simulink model "second"  (R2022b)
settings: Solver=VariableStepAuto  StartTime=0.0  StopTime=10.0  RelTol=1e-3
libraries: spsIGBTDiodeLib x5, simulink x4, spsSeriesRLCBranchLib x4, spsCurrentMeasurementLib x2, spsGroundLib x2, spsVoltageMeasurementLib x2, spsACVoltageSourceLib x1, spsDiodeLib x1, spsPVArrayLib x1, spspowerguiLib x1
settings Model: Creator=Xheng  LastModifiedBy=Xheng

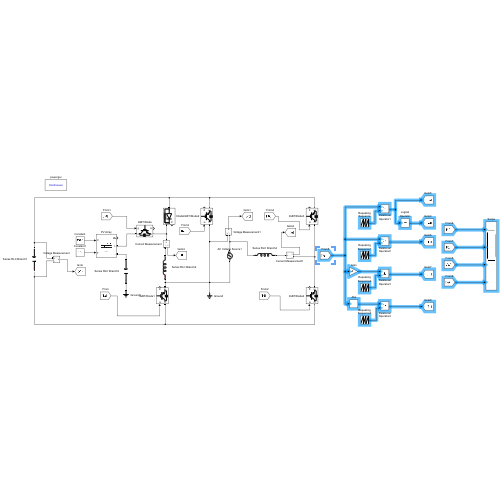
[thumbnail: Simulink's stored preview of the top-level diagram]
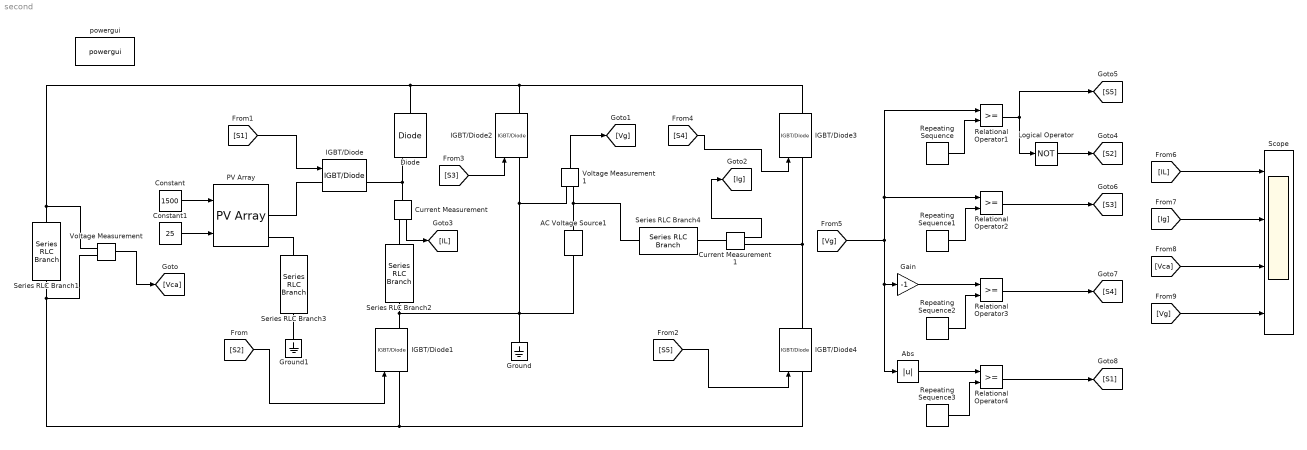
== system second ==
  AC Voltage Source1 : spsACVoltageSourceLib/AC Voltage Source  Amplitude=100  Phase=0  Frequency=60  SampleTime=0  Measurements=None  BusType=swing  Pref=10e3  Qref=0  Qmin=-inf  Qmax=+inf
  Abs : Abs  SaturateOnIntegerOverflow=off
  Constant : Constant  Value=1500
  Constant1 : Constant  Value=25
  Current Measurement : spsCurrentMeasurementLib/Current Measurement  PhasorSimulation=off  OutputType=Complex  PSBequivalent=0
  Current Measurement1 : spsCurrentMeasurementLib/Current Measurement  PhasorSimulation=off  OutputType=Complex  PSBequivalent=0
  Diode : spsDiodeLib/Diode  Ron=0.001  Lon=0  Vf=0.8  IC=0  UseSnubber=0  Rs=500  Cs=250e-9  Measurements=on
  Gain : Gain  Gain=-1
  Ground : spsGroundLib/Ground  LConnTagsString=a
  Ground1 : spsGroundLib/Ground  LConnTagsString=a
  IGBT/Diode{,1..4} (5 alike) : spsIGBTDiodeLib/IGBT//Diode  Ron=1e-3  Rs=1e5  Cs=inf  Measurements=on
  Logical Operator : Logic  Operator=NOT  AllPortsSameDT=off  OutDataTypeStr=boolean
  PV Array : spsPVArrayLib/PV Array  Npar=40  Nser=10  PlotType=array @ 1000 W/m2 & specified temperatures  S_vec="[ 1000  500  100 ]"  Temp_C_vec="[ 45 25  ]"  ModuleName=User-defined  PlotWhenSelected=off  Pm=213.15  Ncell=60  Voc=36.3  Isc=7.84  Vm=29  Im=7.35  beta_Voc_pc=-0.36099  alpha_Isc_pc=0.102  beta_Voc=-0.13104  alpha_Isc=0.0079968  IL=7.8654  I0=2.9273e-10  nI=0.98119  Rsh=313.0553  Rs=0.39381  RobustModel=off  RobustCellTemperature=313.3991  BAL=on  Tc=1e-6  Tfilter=5e-5
  Relational Operator{1..4} (4 alike) : RelationalOperator  OutDataTypeStr=boolean  RndMeth=Simplest  InputSameDT=off
  Repeating Sequence{,1..3} (4 alike) : simulink/Sources/Repeating Sequence  rep_seq_t=[0 2]  rep_seq_y=[0 2]
  Scope : Scope  NumInputPorts=4
  Series RLC Branch1 : spsSeriesRLCBranchLib/Series RLC Branch  LConnTagsString=__new0  RConnTagsString=__new0  BranchType=C  Resistance=1  Inductance=1e-3  SetiL0=off  InitialCurrent=0  Capacitance=50e-6  Setx0=off  InitialVoltage=0  Measurements=None
  Series RLC Branch2 : spsSeriesRLCBranchLib/Series RLC Branch  LConnTagsString=__new0  RConnTagsString=__new0  BranchType=L  Resistance=1  Inductance=115e-6  SetiL0=off  InitialCurrent=0  Capacitance=1e-6  Setx0=off  InitialVoltage=0  Measurements=None
  Series RLC Branch3 : spsSeriesRLCBranchLib/Series RLC Branch  LConnTagsString=__new0  RConnTagsString=__new0  BranchType=C  Resistance=1  Inductance=1e-3  SetiL0=off  InitialCurrent=0  Capacitance=50e-6  Setx0=off  InitialVoltage=0  Measurements=None
  Series RLC Branch4 : spsSeriesRLCBranchLib/Series RLC Branch  LConnTagsString=__new0  RConnTagsString=__new0  BranchType=L  Resistance=1  Inductance=115e-6  SetiL0=off  InitialCurrent=0  Capacitance=1e-6  Setx0=off  InitialVoltage=0  Measurements=None
  Voltage Measurement : spsVoltageMeasurementLib/Voltage Measurement  PhasorSimulation=off  OutputType=Complex  PSBequivalent=0
  Voltage Measurement1 : spsVoltageMeasurementLib/Voltage Measurement  PhasorSimulation=off  OutputType=Complex  PSBequivalent=0
  powergui : spspowerguiLib/powergui  Priority=1  SimulationMode=Continuous  SampleTime=50e-6  frequency=60  Iterations=50  frequencyindice=60  Pbase=100e6  ErrMax=1e-4  UnitsV=kV  UnitsW=MW  buscounter=0  FunctionMessages=off  echomessages=off  EnableUseOfTLC=off  CurrentSourceSwitches=off  DisableSnubberDevices=off  DisableRonSwitches=off  DisableVfSwitches=off  DisplayEquations=off  AutomaticDiscreteSolvers=off  SolverType=Tustin/Backward Euler (TBE)  Interpol=off  ExternalGateDelay=off  methode=off  Ts=100  x0status=blocks  SPID=on  SwTol=0  HookPort=off  NonlinearTolerance=1e-4  nMaxIteration=100  ContinueOnMaxIteration=off  RestoreLinks=warning  ResistiveCurrentMeasurement=off  Frange=[0:2:500]  Ylog=off  Xlog=on  ShowGrid=off  save=off  variable=ZData  structure=0  ZoomFFT=off  StartTime=0.0  cycles=1  DisplayStyle=1  fundamental=60  FreqAxis=off  MaxFrequency=1000  frequencyindicesteady=1  RmsSteady=1  display=off
  wires:
  Constant1/1 -> PV Array/2
  Constant/1 -> PV Array/1
  Voltage Measurement/1 -> [Vca]
  Voltage Measurement1/1 -> [Vg]
  Current Measurement1/1 -> [Ig]
  Current Measurement/1 -> [IL]
  [S1] -> IGBT/Diode/1
  [S2] -> IGBT/Diode1/1
  [S5] -> IGBT/Diode4/1
  [S3] -> IGBT/Diode2/1
  [S4] -> IGBT/Diode3/1
  Logical Operator/1 -> [S2]
  Relational Operator1/1 -> Logical Operator/1, [S5]
  [Vg] -> Abs/1, Gain/1, Relational Operator1/1, Relational Operator2/1
  Repeating Sequence/1 -> Relational Operator1/2
  Repeating Sequence1/1 -> Relational Operator2/2
  Relational Operator2/1 -> [S3]
  Repeating Sequence2/1 -> Relational Operator3/2
  Relational Operator3/1 -> [S4]
  Repeating Sequence3/1 -> Relational Operator4/2
  Relational Operator4/1 -> [S1]
  Gain/1 -> Relational Operator3/1
  Abs/1 -> Relational Operator4/1
  [IL] -> Scope/1
  [Ig] -> Scope/2
  [Vca] -> Scope/3
  [Vg] -> Scope/4
  connections:
  PV Array/RConn1 -- IGBT/Diode/LConn1
  IGBT/Diode/RConn1 -- Diode/RConn1 -- Current Measurement/LConn1
  Diode/LConn1 -- IGBT/Diode3/RConn1 -- IGBT/Diode2/RConn1 -- Voltage Measurement/LConn1 -- Series RLC Branch1/RConn1
  Voltage Measurement/LConn2 -- IGBT/Diode1/LConn1 -- IGBT/Diode4/LConn1 -- Series RLC Branch1/LConn1
  Current Measurement/RConn1 -- Series RLC Branch2/RConn1
  Series RLC Branch2/LConn1 -- Voltage Measurement1/LConn1 -- IGBT/Diode2/LConn1 -- Ground/LConn1 -- AC Voltage Source1/LConn1 -- IGBT/Diode1/RConn1
  PV Array/RConn2 -- Series RLC Branch3/RConn1
  Current Measurement1/LConn1 -- Series RLC Branch4/RConn1
  Current Measurement1/RConn1 -- IGBT/Diode3/LConn1 -- IGBT/Diode4/RConn1
  AC Voltage Source1/RConn1 -- Series RLC Branch4/LConn1 -- Voltage Measurement1/LConn2
  Ground1/LConn1 -- Series RLC Branch3/LConn1
